simulink model "three_phase_dab"  (R2025a)
settings: Solver=ode1be  StartTime=0.0  StopTime=simlength  FixedStep=ts_sim  MaxStep=ts_sim
undefined symbols (not defined in the file or in its folder): Adrso, Aresd, Bresd, Cresd, Crso, dead_time, DThs_init, fPWM_INV, fPWM_ZVS, freq, frequency_grid, I_FS, Iout_dc_nom, ki_i_inv, ki_i_zvs, ki_pll, ki_v_inv, ki_v_zvs, kp_i_inv, kp_i_zvs, kp_pll, kp_v_inv, kp_v_zvs, Ldrso, magnitude, number_of_cells, Q, q1Kalman, q1kalman, q2Kalman, q2kalman, q3Kalman, rKalman, Rkalman, Tambient, tc, ts_dab, ts_inv, ts_zvs, tsample, V_FS, Vout_dc_nom, w, weigth
libraries: fl_lib x136, nesl_utility x98, ee_lib x21, cstblocks x7, lithium_ion_cell_lib x1, simulink x1, single_phase_transformer_lib x1
(part 2 of 7)

== system three_phase_dab/dab_modA/dab_ctrl/vi ctrl ==
  iout : Inport
  vout : Inport  Port=2
  vout_ref : Inport  Port=3
  Constant : Constant  Value=Iout_dc_nom
  Iout Ctrl : Subsystem
  Min : MinMax  Inputs=2
  To Workspace1 : ToWorkspace  VariableName=phase_ctrl_out_modA_sim  SampleTime=ts_zvs
      settings: MaxDataPoints=Ns_zvs
  To Workspace2 : ToWorkspace  VariableName=pid_ctrlv_out_modA_sim  SampleTime=ts_zvs
      settings: MaxDataPoints=Ns_zvs
  To Workspace3 : ToWorkspace  VariableName=pid_ctrli_out_modA_sim  SampleTime=ts_zvs
      settings: MaxDataPoints=Ns_zvs
  Unit Delay2 : UnitDelay  SampleTime=ts_zvs  HasFrameUpgradeWarning=on
  Vout Ctrl : Subsystem
  zvs_ctrl : Scope  NumInputPorts=2
      settings: SampleTime=tc  ActiveDisplayYMinimum=-1.16562  ActiveDisplayYMaximum=0.4906
  phase_displacement : Outport
  wires:
  Unit Delay2/1 -> phase_displacement/1, To Workspace1/1
  iout/1 -> Iout Ctrl/2(iout)
  vout_ref/1 -> Vout Ctrl/1(vout_ref)
  vout/1 -> Vout Ctrl/2(vout)
  Vout Ctrl/1(ctrlv_out) -> zvs_ctrl/1, Unit Delay2/1, To Workspace2/1  "u_ctrl_out"
  Constant/1 -> Iout Ctrl/1(iout_ref)
  Iout Ctrl/1(ctrli_out) -> zvs_ctrl/2, To Workspace3/1, Min/2  "i_ctrl_out"

== system three_phase_dab/dab_modA/dc//dc with galvanic isolation/stage-1 ==
  gate_commands : Inport
  Current Sensor : fl_lib/Electrical/Electrical Sensors/Current Sensor
  PS-Simulink Converter1 : nesl_utility/PS-Simulink Converter  PhysicalDomain=network_engine_domain  SubClassName=ps_output  LeftPortType=input  RightPortType=output  PseudoPeriodic=off  Frequencies=[]  VectorFormat=1-D array  Unit=A  AffineConversion=on
  h-bridge_thermal : Subsystem  Commented=on
  h-ideal : Subsystem  Commented=on
  h-mosfet : Subsystem
  uac_1(+) : PMIOPort  Side=Left
  uac_1(-) : PMIOPort  Port=2  Side=Left
  Udc(+) : PMIOPort  Port=3  Side=Right
  Udc(-) : PMIOPort  Port=4  Side=Right
  tag scope: dc_bus_terminal_current_inverter=global
  wires:
  gate_commands/1 -> h-mosfet/1(gate_commands)
  PS-Simulink Converter1/1 -> [dc_bus_terminal_current_inverter]  "idc"
  connections:
  h-mosfet/LConn1 -- uac_1(+)/RConn1
  h-mosfet/LConn2 -- uac_1(-)/RConn1
  h-mosfet/RConn2 -- Udc(-)/RConn1
  Current Sensor/LConn1 -- Udc(+)/RConn1
  h-mosfet/RConn1 -- Current Sensor/RConn2
  PS-Simulink Converter1/LConn1 -- Current Sensor/RConn1

== system three_phase_dab/dab_modA/dc//dc with galvanic isolation/stage-2 ==
  Current Sensor1 : fl_lib/Electrical/Electrical Sensors/Current Sensor
  PS-Simulink Converter2 : nesl_utility/PS-Simulink Converter  PhysicalDomain=network_engine_domain  SubClassName=ps_output  LeftPortType=input  RightPortType=output  PseudoPeriodic=off  Frequencies=[]  VectorFormat=1-D array  Unit=A  AffineConversion=on
  hf_trafo_center_tap_ss : Subsystem
  uac_1(+) : PMIOPort  Side=Left
  uac_2(+) : PMIOPort  Port=2  Side=Right
  uac_1(-) : PMIOPort  Port=3  Side=Left
  uac_2(-) : PMIOPort  Port=4  Side=Right
  connections:
  Current Sensor1/RConn2 -- uac_2(+)/RConn1
  PS-Simulink Converter2/LConn1 -- Current Sensor1/RConn1
  hf_trafo_center_tap_ss/LConn1 -- uac_1(+)/RConn1
  hf_trafo_center_tap_ss/RConn1 -- Current Sensor1/LConn1
  hf_trafo_center_tap_ss/LConn2 -- uac_1(-)/RConn1
  hf_trafo_center_tap_ss/RConn2 -- uac_2(-)/RConn1

== system three_phase_dab/dab_modA/dc//dc with galvanic isolation/stage-3 ==
  gate_commands : Inport
  CFu_dc : fl_lib/Electrical/Electrical Elements/Capacitor  c=CFu_dc F  r=RCFu_dc_internal Ohm  g=0 1/Ohm  i_specify=off  i_priority=None  i=0 A  i_nominal_specify=off  i_nominal_value=1  i_nominal_unit=A  v_specify=off  v_priority=None  v=0 V  v_nominal_specify=off  v_nominal_value=1  v_nominal_unit=V  vc_specify=off  vc_priority=High  vc=0 V  vc_nominal_specify=off  vc_nominal_value=1  vc_nominal_unit=V
  Current Sensor : fl_lib/Electrical/Electrical Sensors/Current Sensor
  Current Sensor2 : fl_lib/Electrical/Electrical Sensors/Current Sensor
  PS-Simulink Converter1 : nesl_utility/PS-Simulink Converter  PhysicalDomain=network_engine_domain  SubClassName=ps_output  LeftPortType=input  RightPortType=output  PseudoPeriodic=off  Frequencies=[]  VectorFormat=1-D array  Unit=A  AffineConversion=on
  PS-Simulink Converter6 : nesl_utility/PS-Simulink Converter  PhysicalDomain=network_engine_domain  SubClassName=ps_output  LeftPortType=input  RightPortType=output  PseudoPeriodic=off  Frequencies=[]  VectorFormat=1-D array  Unit=A  AffineConversion=on
  PS-Simulink Converter8 : nesl_utility/PS-Simulink Converter  PhysicalDomain=network_engine_domain  SubClassName=ps_output  LeftPortType=input  RightPortType=output  PseudoPeriodic=off  Frequencies=[]  VectorFormat=1-D array  Unit=V  AffineConversion=on
  Voltage Sensor4 : fl_lib/Electrical/Electrical Sensors/Voltage Sensor
  h-mosfet : Subsystem
  uac_1(+) : PMIOPort  Side=Left
  uac_1(-) : PMIOPort  Port=2  Side=Left
  udc(+) : PMIOPort  Port=3  Side=Right
  udc(-) : PMIOPort  Port=4  Side=Right
  tag scope: CFu_dc_current=global, CFu_dc_voltage=global
  wires:
  gate_commands/1 -> h-mosfet/1(gate_commands)
  PS-Simulink Converter6/1 -> [CFu_dc_current]  "i_Ls"
  PS-Simulink Converter8/1 -> [CFu_dc_voltage]  "CFu_dc_voltage"
  connections:
  h-mosfet/RConn1 -- Current Sensor/LConn1 -- CFu_dc/LConn1
  Voltage Sensor4/LConn1 -- udc(+)/RConn1 -- Current Sensor/RConn2
  h-mosfet/RConn2 -- Current Sensor2/RConn2 -- udc(-)/RConn1 -- Voltage Sensor4/RConn2
  h-mosfet/LConn2 -- uac_1(-)/RConn1
  h-mosfet/LConn1 -- uac_1(+)/RConn1
  Voltage Sensor4/RConn1 -- PS-Simulink Converter8/LConn1
  PS-Simulink Converter6/LConn1 -- Current Sensor2/RConn1
  CFu_dc/RConn1 -- Current Sensor2/LConn1
  Current Sensor/RConn1 -- PS-Simulink Converter1/LConn1

== system three_phase_dab/inverter_modA/single phase inverter/HBridgeIdeal ==
  gate_commands : Inport
  Bus Selector : BusSelector  OutputSignals=gate_cmd_Q1,gate_cmd_Q2,gate_cmd_Q3,gate_cmd_Q4
  Simulink-PS Converter{,1..3} (4 alike) : nesl_utility/Simulink-PS Converter  PhysicalDomain=network_engine_domain  SubClassName=ps_input  LeftPortType=input  RightPortType=output  PseudoPeriodic=off  Frequencies=[]  NoiseDistribution=none  NoiseParameters=[]  Unit=1  AffineConversion=on  FilteringAndDerivatives=provide  SimscapeFilterOrder=1  InputFilterTimeConstant=0.001  UdotUserProvided=0
  switch_1 : Subsystem
      settings: PortSchema="{\"entries\":[{\"content\":{\"sides\":[{\"content\":{\"connectorIds\":[\"LConn1\"]},\"type\":\"ConnectorPlacement.EquallySpacedRectSide\",\"uuid\":\"9277da8d-d460-43e6-8478-dd662f15d226\"},{\"content\":{\"connectorIds\":[],\"side\":\"RIGHT\"},\"type\":\"ConnectorPlacement.EquallySpacedRectSide\",\"uuid\":\"a7ece396-f1d9-4f4f-a05b-db1fc65d6e1d\"},{\"content\":{\"connectorIds\":[\"LConn2\"],\"side\":\"TOP\"},\"type\":\"ConnectorPlacement.EquallySpacedRectSide\",\"uuid\":\"fdd70777-e9cf-4317-afb6-cae87f75d5b0\"},{\"content\":{\"connectorIds\":[\"RConn1\"],\"side\":\"BOTTOM\"},\"type\":\"ConnectorPlacement.EquallySpacedRectSide\",\"uuid\":\"2353ed68-b1a1-4775-9ca9-31e268d5443b\"}]},\"type\":\"ConnectorPlacement.EquallySpacedConnector\",\"uuid\":\"d5479f4c-4e65-4791-adcb-73df11f88590\"}],\"packageUris\":[\"http://schema.mathworks.com/mf0/Connector/R2020b\"],\"version\":\"1.0\"}"
  switch_2 : Subsystem
      settings: PortSchema="{\"entries\":[{\"content\":{\"sides\":[{\"content\":{\"connectorIds\":[\"LConn1\"]},\"type\":\"ConnectorPlacement.EquallySpacedRectSide\",\"uuid\":\"9277da8d-d460-43e6-8478-dd662f15d226\"},{\"content\":{\"connectorIds\":[],\"side\":\"RIGHT\"},\"type\":\"ConnectorPlacement.EquallySpacedRectSide\",\"uuid\":\"a7ece396-f1d9-4f4f-a05b-db1fc65d6e1d\"},{\"content\":{\"connectorIds\":[\"LConn2\"],\"side\":\"TOP\"},\"type\":\"ConnectorPlacement.EquallySpacedRectSide\",\"uuid\":\"fdd70777-e9cf-4317-afb6-cae87f75d5b0\"},{\"content\":{\"connectorIds\":[\"RConn1\"],\"side\":\"BOTTOM\"},\"type\":\"ConnectorPlacement.EquallySpacedRectSide\",\"uuid\":\"2353ed68-b1a1-4775-9ca9-31e268d5443b\"}]},\"type\":\"ConnectorPlacement.EquallySpacedConnector\",\"uuid\":\"d5479f4c-4e65-4791-adcb-73df11f88590\"}],\"packageUris\":[\"http://schema.mathworks.com/mf0/Connector/R2020b\"],\"version\":\"1.0\"}"
  switch_3 : Subsystem
      settings: PortSchema="{\"entries\":[{\"content\":{\"sides\":[{\"content\":{\"connectorIds\":[\"LConn1\"]},\"type\":\"ConnectorPlacement.EquallySpacedRectSide\",\"uuid\":\"9277da8d-d460-43e6-8478-dd662f15d226\"},{\"content\":{\"connectorIds\":[],\"side\":\"RIGHT\"},\"type\":\"ConnectorPlacement.EquallySpacedRectSide\",\"uuid\":\"a7ece396-f1d9-4f4f-a05b-db1fc65d6e1d\"},{\"content\":{\"connectorIds\":[\"LConn2\"],\"side\":\"TOP\"},\"type\":\"ConnectorPlacement.EquallySpacedRectSide\",\"uuid\":\"fdd70777-e9cf-4317-afb6-cae87f75d5b0\"},{\"content\":{\"connectorIds\":[\"RConn1\"],\"side\":\"BOTTOM\"},\"type\":\"ConnectorPlacement.EquallySpacedRectSide\",\"uuid\":\"2353ed68-b1a1-4775-9ca9-31e268d5443b\"}]},\"type\":\"ConnectorPlacement.EquallySpacedConnector\",\"uuid\":\"d5479f4c-4e65-4791-adcb-73df11f88590\"}],\"packageUris\":[\"http://schema.mathworks.com/mf0/Connector/R2020b\"],\"version\":\"1.0\"}"
  switch_4 : Subsystem
      settings: PortSchema="{\"entries\":[{\"content\":{\"sides\":[{\"content\":{\"connectorIds\":[\"LConn1\"]},\"type\":\"ConnectorPlacement.EquallySpacedRectSide\",\"uuid\":\"9277da8d-d460-43e6-8478-dd662f15d226\"},{\"content\":{\"connectorIds\":[],\"side\":\"RIGHT\"},\"type\":\"ConnectorPlacement.EquallySpacedRectSide\",\"uuid\":\"a7ece396-f1d9-4f4f-a05b-db1fc65d6e1d\"},{\"content\":{\"connectorIds\":[\"LConn2\"],\"side\":\"TOP\"},\"type\":\"ConnectorPlacement.EquallySpacedRectSide\",\"uuid\":\"fdd70777-e9cf-4317-afb6-cae87f75d5b0\"},{\"content\":{\"connectorIds\":[\"RConn1\"],\"side\":\"BOTTOM\"},\"type\":\"ConnectorPlacement.EquallySpacedRectSide\",\"uuid\":\"2353ed68-b1a1-4775-9ca9-31e268d5443b\"}]},\"type\":\"ConnectorPlacement.EquallySpacedConnector\",\"uuid\":\"d5479f4c-4e65-4791-adcb-73df11f88590\"}],\"packageUris\":[\"http://schema.mathworks.com/mf0/Connector/R2020b\"],\"version\":\"1.0\"}"
  C : PMIOPort  Side=Left
  E : PMIOPort  Port=2  Side=Right
  C1 : PMIOPort  Port=3  Side=Right
  E1 : PMIOPort  Port=4  Side=Left
  wires:
  [gate_Q3] -> Simulink-PS Converter2/1
  Bus Selector/2 -> [gate_Q2]  "<gate_cmd_Q2>"
  Bus Selector/1 -> [gate_Q1]  "<gate_cmd_Q1>"
  Bus Selector/3 -> [gate_Q3]  "<gate_cmd_Q3>"
  [gate_Q4] -> Simulink-PS Converter3/1
  [gate_Q2] -> Simulink-PS Converter1/1
  [gate_Q1] -> Simulink-PS Converter/1
  Bus Selector/4 -> [gate_Q4]  "<gate_cmd_Q4>"
  gate_commands/1 -> Bus Selector/1
  connections:
  switch_1/LConn1 -- Simulink-PS Converter/RConn1
  switch_3/LConn2 -- C/RConn1 -- switch_1/LConn2
  switch_4/RConn1 -- E1/RConn1 -- switch_2/RConn1
  switch_2/LConn2 -- switch_1/RConn1 -- E/RConn1
  switch_3/LConn1 -- Simulink-PS Converter2/RConn1
  switch_3/RConn1 -- switch_4/LConn2 -- C1/RConn1
  switch_2/LConn1 -- Simulink-PS Converter1/RConn1
  switch_4/LConn1 -- Simulink-PS Converter3/RConn1

== system three_phase_dab/inverter_modA/single phase inverter/HBridgeMosfet ==
  gate_commands : Inport
  Bus Selector : BusSelector  OutputSignals=gate_cmd_Q1,gate_cmd_Q2,gate_cmd_Q3,gate_cmd_Q4
  Simulink-PS Converter{,1..3} (4 alike) : nesl_utility/Simulink-PS Converter  PhysicalDomain=network_engine_domain  SubClassName=ps_input  LeftPortType=input  RightPortType=output  PseudoPeriodic=off  Frequencies=[]  NoiseDistribution=none  NoiseParameters=[]  Unit=V  AffineConversion=off  FilteringAndDerivatives=provide  SimscapeFilterOrder=1  InputFilterTimeConstant=0.001  UdotUserProvided=0
  mosfet_1 : Subsystem
      settings: PortSchema="{\"entries\":[{\"content\":{\"sides\":[{\"content\":{\"connectorIds\":[\"LConn1\"]},\"type\":\"ConnectorPlacement.EquallySpacedRectSide\",\"uuid\":\"9277da8d-d460-43e6-8478-dd662f15d226\"},{\"content\":{\"connectorIds\":[],\"side\":\"RIGHT\"},\"type\":\"ConnectorPlacement.EquallySpacedRectSide\",\"uuid\":\"a7ece396-f1d9-4f4f-a05b-db1fc65d6e1d\"},{\"content\":{\"connectorIds\":[\"LConn2\"],\"side\":\"TOP\"},\"type\":\"ConnectorPlacement.EquallySpacedRectSide\",\"uuid\":\"fdd70777-e9cf-4317-afb6-cae87f75d5b0\"},{\"content\":{\"connectorIds\":[\"RConn1\"],\"side\":\"BOTTOM\"},\"type\":\"ConnectorPlacement.EquallySpacedRectSide\",\"uuid\":\"2353ed68-b1a1-4775-9ca9-31e268d5443b\"}]},\"type\":\"ConnectorPlacement.EquallySpacedConnector\",\"uuid\":\"d5479f4c-4e65-4791-adcb-73df11f88590\"}],\"packageUris\":[\"http://schema.mathworks.com/mf0/Connector/R2020b\"],\"version\":\"1.0\"}"
  mosfet_2 : Subsystem
      settings: PortSchema="{\"entries\":[{\"content\":{\"sides\":[{\"content\":{\"connectorIds\":[\"LConn1\"]},\"type\":\"ConnectorPlacement.EquallySpacedRectSide\",\"uuid\":\"9277da8d-d460-43e6-8478-dd662f15d226\"},{\"content\":{\"connectorIds\":[],\"side\":\"RIGHT\"},\"type\":\"ConnectorPlacement.EquallySpacedRectSide\",\"uuid\":\"a7ece396-f1d9-4f4f-a05b-db1fc65d6e1d\"},{\"content\":{\"connectorIds\":[\"LConn2\"],\"side\":\"TOP\"},\"type\":\"ConnectorPlacement.EquallySpacedRectSide\",\"uuid\":\"fdd70777-e9cf-4317-afb6-cae87f75d5b0\"},{\"content\":{\"connectorIds\":[\"RConn1\"],\"side\":\"BOTTOM\"},\"type\":\"ConnectorPlacement.EquallySpacedRectSide\",\"uuid\":\"2353ed68-b1a1-4775-9ca9-31e268d5443b\"}]},\"type\":\"ConnectorPlacement.EquallySpacedConnector\",\"uuid\":\"d5479f4c-4e65-4791-adcb-73df11f88590\"}],\"packageUris\":[\"http://schema.mathworks.com/mf0/Connector/R2020b\"],\"version\":\"1.0\"}"
  mosfet_3 : Subsystem
      settings: PortSchema="{\"entries\":[{\"content\":{\"sides\":[{\"content\":{\"connectorIds\":[\"LConn1\"]},\"type\":\"ConnectorPlacement.EquallySpacedRectSide\",\"uuid\":\"9277da8d-d460-43e6-8478-dd662f15d226\"},{\"content\":{\"connectorIds\":[],\"side\":\"RIGHT\"},\"type\":\"ConnectorPlacement.EquallySpacedRectSide\",\"uuid\":\"a7ece396-f1d9-4f4f-a05b-db1fc65d6e1d\"},{\"content\":{\"connectorIds\":[\"LConn2\"],\"side\":\"TOP\"},\"type\":\"ConnectorPlacement.EquallySpacedRectSide\",\"uuid\":\"fdd70777-e9cf-4317-afb6-cae87f75d5b0\"},{\"content\":{\"connectorIds\":[\"RConn1\"],\"side\":\"BOTTOM\"},\"type\":\"ConnectorPlacement.EquallySpacedRectSide\",\"uuid\":\"2353ed68-b1a1-4775-9ca9-31e268d5443b\"}]},\"type\":\"ConnectorPlacement.EquallySpacedConnector\",\"uuid\":\"d5479f4c-4e65-4791-adcb-73df11f88590\"}],\"packageUris\":[\"http://schema.mathworks.com/mf0/Connector/R2020b\"],\"version\":\"1.0\"}"
  mosfet_4 : Subsystem
      settings: PortSchema="{\"entries\":[{\"content\":{\"sides\":[{\"content\":{\"connectorIds\":[\"LConn1\"]},\"type\":\"ConnectorPlacement.EquallySpacedRectSide\",\"uuid\":\"9277da8d-d460-43e6-8478-dd662f15d226\"},{\"content\":{\"connectorIds\":[],\"side\":\"RIGHT\"},\"type\":\"ConnectorPlacement.EquallySpacedRectSide\",\"uuid\":\"a7ece396-f1d9-4f4f-a05b-db1fc65d6e1d\"},{\"content\":{\"connectorIds\":[\"LConn2\"],\"side\":\"TOP\"},\"type\":\"ConnectorPlacement.EquallySpacedRectSide\",\"uuid\":\"fdd70777-e9cf-4317-afb6-cae87f75d5b0\"},{\"content\":{\"connectorIds\":[\"RConn1\"],\"side\":\"BOTTOM\"},\"type\":\"ConnectorPlacement.EquallySpacedRectSide\",\"uuid\":\"2353ed68-b1a1-4775-9ca9-31e268d5443b\"}]},\"type\":\"ConnectorPlacement.EquallySpacedConnector\",\"uuid\":\"d5479f4c-4e65-4791-adcb-73df11f88590\"}],\"packageUris\":[\"http://schema.mathworks.com/mf0/Connector/R2020b\"],\"version\":\"1.0\"}"
  C : PMIOPort  Side=Left
  E : PMIOPort  Port=2  Side=Right
  C1 : PMIOPort  Port=3  Side=Right
  E1 : PMIOPort  Port=4  Side=Left
  wires:
  [gate_Q3] -> Simulink-PS Converter2/1
  Bus Selector/2 -> [gate_Q2]  "<gate_cmd_Q2>"
  Bus Selector/1 -> [gate_Q1]  "<gate_cmd_Q1>"
  Bus Selector/3 -> [gate_Q3]  "<gate_cmd_Q3>"
  [gate_Q4] -> Simulink-PS Converter3/1
  [gate_Q2] -> Simulink-PS Converter1/1
  [gate_Q1] -> Simulink-PS Converter/1
  Bus Selector/4 -> [gate_Q4]  "<gate_cmd_Q4>"
  gate_commands/1 -> Bus Selector/1
  connections:
  mosfet_1/LConn1 -- Simulink-PS Converter/RConn1
  C/RConn1 -- mosfet_3/LConn2 -- mosfet_1/LConn2
  E1/RConn1 -- mosfet_4/RConn1 -- mosfet_2/RConn1
  E/RConn1 -- mosfet_2/LConn2 -- mosfet_1/RConn1
  mosfet_3/LConn1 -- Simulink-PS Converter2/RConn1
  C1/RConn1 -- mosfet_4/LConn2 -- mosfet_3/RConn1
  mosfet_2/LConn1 -- Simulink-PS Converter1/RConn1
  mosfet_4/LConn1 -- Simulink-PS Converter3/RConn1

== system three_phase_dab/inverter_modA/single phase inverter/HBridgeThermal ==
  gate_commands : Inport
  Bus Selector : BusSelector  OutputSignals=gate_cmd_Q1,gate_cmd_Q2,gate_cmd_Q3,gate_cmd_Q4
  Simulink-PS Converter{,1..3} (4 alike) : nesl_utility/Simulink-PS Converter  PhysicalDomain=network_engine_domain  SubClassName=ps_input  LeftPortType=input  RightPortType=output  PseudoPeriodic=off  Frequencies=[]  NoiseDistribution=none  NoiseParameters=[]  Unit=V  AffineConversion=off  FilteringAndDerivatives=provide  SimscapeFilterOrder=1  InputFilterTimeConstant=0.001  UdotUserProvided=0
  mosfet_thermal_1 : Subsystem
      settings: PortSchema="{\"entries\":[{\"content\":{\"sides\":[{\"content\":{\"connectorIds\":[\"LConn1\"]},\"type\":\"ConnectorPlacement.EquallySpacedRectSide\",\"uuid\":\"9277da8d-d460-43e6-8478-dd662f15d226\"},{\"content\":{\"connectorIds\":[],\"side\":\"RIGHT\"},\"type\":\"ConnectorPlacement.EquallySpacedRectSide\",\"uuid\":\"a7ece396-f1d9-4f4f-a05b-db1fc65d6e1d\"},{\"content\":{\"connectorIds\":[\"LConn2\"],\"side\":\"TOP\"},\"type\":\"ConnectorPlacement.EquallySpacedRectSide\",\"uuid\":\"fdd70777-e9cf-4317-afb6-cae87f75d5b0\"},{\"content\":{\"connectorIds\":[\"RConn1\"],\"side\":\"BOTTOM\"},\"type\":\"ConnectorPlacement.EquallySpacedRectSide\",\"uuid\":\"2353ed68-b1a1-4775-9ca9-31e268d5443b\"}]},\"type\":\"ConnectorPlacement.EquallySpacedConnector\",\"uuid\":\"d5479f4c-4e65-4791-adcb-73df11f88590\"}],\"packageUris\":[\"http://schema.mathworks.com/mf0/Connector/R2020b\"],\"version\":\"1.0\"}"
  mosfet_thermal_2 : Subsystem
      settings: PortSchema="{\"entries\":[{\"content\":{\"sides\":[{\"content\":{\"connectorIds\":[\"LConn1\"]},\"type\":\"ConnectorPlacement.EquallySpacedRectSide\",\"uuid\":\"9277da8d-d460-43e6-8478-dd662f15d226\"},{\"content\":{\"connectorIds\":[],\"side\":\"RIGHT\"},\"type\":\"ConnectorPlacement.EquallySpacedRectSide\",\"uuid\":\"a7ece396-f1d9-4f4f-a05b-db1fc65d6e1d\"},{\"content\":{\"connectorIds\":[\"LConn2\"],\"side\":\"TOP\"},\"type\":\"ConnectorPlacement.EquallySpacedRectSide\",\"uuid\":\"fdd70777-e9cf-4317-afb6-cae87f75d5b0\"},{\"content\":{\"connectorIds\":[\"RConn1\"],\"side\":\"BOTTOM\"},\"type\":\"ConnectorPlacement.EquallySpacedRectSide\",\"uuid\":\"2353ed68-b1a1-4775-9ca9-31e268d5443b\"}]},\"type\":\"ConnectorPlacement.EquallySpacedConnector\",\"uuid\":\"d5479f4c-4e65-4791-adcb-73df11f88590\"}],\"packageUris\":[\"http://schema.mathworks.com/mf0/Connector/R2020b\"],\"version\":\"1.0\"}"
  mosfet_thermal_3 : Subsystem
      settings: PortSchema="{\"entries\":[{\"content\":{\"sides\":[{\"content\":{\"connectorIds\":[\"LConn1\"]},\"type\":\"ConnectorPlacement.EquallySpacedRectSide\",\"uuid\":\"9277da8d-d460-43e6-8478-dd662f15d226\"},{\"content\":{\"connectorIds\":[],\"side\":\"RIGHT\"},\"type\":\"ConnectorPlacement.EquallySpacedRectSide\",\"uuid\":\"a7ece396-f1d9-4f4f-a05b-db1fc65d6e1d\"},{\"content\":{\"connectorIds\":[\"LConn2\"],\"side\":\"TOP\"},\"type\":\"ConnectorPlacement.EquallySpacedRectSide\",\"uuid\":\"fdd70777-e9cf-4317-afb6-cae87f75d5b0\"},{\"content\":{\"connectorIds\":[\"RConn1\"],\"side\":\"BOTTOM\"},\"type\":\"ConnectorPlacement.EquallySpacedRectSide\",\"uuid\":\"2353ed68-b1a1-4775-9ca9-31e268d5443b\"}]},\"type\":\"ConnectorPlacement.EquallySpacedConnector\",\"uuid\":\"d5479f4c-4e65-4791-adcb-73df11f88590\"}],\"packageUris\":[\"http://schema.mathworks.com/mf0/Connector/R2020b\"],\"version\":\"1.0\"}"
  mosfet_thermal_4 : Subsystem
      settings: PortSchema="{\"entries\":[{\"content\":{\"sides\":[{\"content\":{\"connectorIds\":[\"LConn1\"]},\"type\":\"ConnectorPlacement.EquallySpacedRectSide\",\"uuid\":\"9277da8d-d460-43e6-8478-dd662f15d226\"},{\"content\":{\"connectorIds\":[],\"side\":\"RIGHT\"},\"type\":\"ConnectorPlacement.EquallySpacedRectSide\",\"uuid\":\"a7ece396-f1d9-4f4f-a05b-db1fc65d6e1d\"},{\"content\":{\"connectorIds\":[\"LConn2\"],\"side\":\"TOP\"},\"type\":\"ConnectorPlacement.EquallySpacedRectSide\",\"uuid\":\"fdd70777-e9cf-4317-afb6-cae87f75d5b0\"},{\"content\":{\"connectorIds\":[\"RConn1\"],\"side\":\"BOTTOM\"},\"type\":\"ConnectorPlacement.EquallySpacedRectSide\",\"uuid\":\"2353ed68-b1a1-4775-9ca9-31e268d5443b\"}]},\"type\":\"ConnectorPlacement.EquallySpacedConnector\",\"uuid\":\"d5479f4c-4e65-4791-adcb-73df11f88590\"}],\"packageUris\":[\"http://schema.mathworks.com/mf0/Connector/R2020b\"],\"version\":\"1.0\"}"
  C : PMIOPort  Side=Left
  E : PMIOPort  Port=2  Side=Right
  C1 : PMIOPort  Port=3  Side=Right
  E1 : PMIOPort  Port=4  Side=Left
  wires:
  gate_commands/1 -> Bus Selector/1
  Bus Selector/4 -> [gate_Q4]  "<gate_cmd_Q4>"
  [gate_Q1] -> Simulink-PS Converter/1
  [gate_Q2] -> Simulink-PS Converter1/1
  [gate_Q4] -> Simulink-PS Converter3/1
  Bus Selector/3 -> [gate_Q3]  "<gate_cmd_Q3>"
  Bus Selector/1 -> [gate_Q1]  "<gate_cmd_Q1>"
  Bus Selector/2 -> [gate_Q2]  "<gate_cmd_Q2>"
  [gate_Q3] -> Simulink-PS Converter2/1
  connections:
  mosfet_thermal_4/LConn1 -- Simulink-PS Converter3/RConn1
  mosfet_thermal_2/LConn1 -- Simulink-PS Converter1/RConn1
  C1/RConn1 -- mosfet_thermal_4/LConn2 -- mosfet_thermal_3/RConn1
  mosfet_thermal_3/LConn1 -- Simulink-PS Converter2/RConn1
  E/RConn1 -- mosfet_thermal_1/RConn1 -- mosfet_thermal_2/LConn2
  E1/RConn1 -- mosfet_thermal_4/RConn1 -- mosfet_thermal_2/RConn1
  mosfet_thermal_1/LConn2 -- mosfet_thermal_3/LConn2 -- C/RConn1
  mosfet_thermal_1/LConn1 -- Simulink-PS Converter/RConn1

== system three_phase_dab/inverter_modA/single phase inverter control/acquisition_and_scaling_current ==
  in : Inport
  1/Ti5 : Gain  Gain=1/I_FS  SaturateOnIntegerOverflow=on  OutDataTypeStr=Inherit: Same as input  ParamDataTypeStr=Inherit: Same as input
  Unit Delay4 : UnitDelay  SampleTime=ts_inv  HasFrameUpgradeWarning=on
  Zero-Order Hold1 : ZeroOrderHold  SampleTime=ts_inv
  out : Outport
  wires:
  in/1 -> Zero-Order Hold1/1
  1/Ti5/1 -> Unit Delay4/1
  Zero-Order Hold1/1 -> 1/Ti5/1
  Unit Delay4/1 -> out/1

== system three_phase_dab/inverter_modA/single phase inverter control/acquisition_and_scaling_voltage ==
  in : Inport
  1/Ti1 : Gain  Gain=1/V_FS  SaturateOnIntegerOverflow=on  OutDataTypeStr=Inherit: Same as input  ParamDataTypeStr=Inherit: Same as input
  Unit Delay4 : UnitDelay  SampleTime=ts_inv  HasFrameUpgradeWarning=on
  Zero-Order Hold2 : ZeroOrderHold  SampleTime=ts_inv
  out : Outport
  wires:
  1/Ti1/1 -> Unit Delay4/1
  Zero-Order Hold2/1 -> 1/Ti1/1
  Unit Delay4/1 -> out/1
  in/1 -> Zero-Order Hold2/1

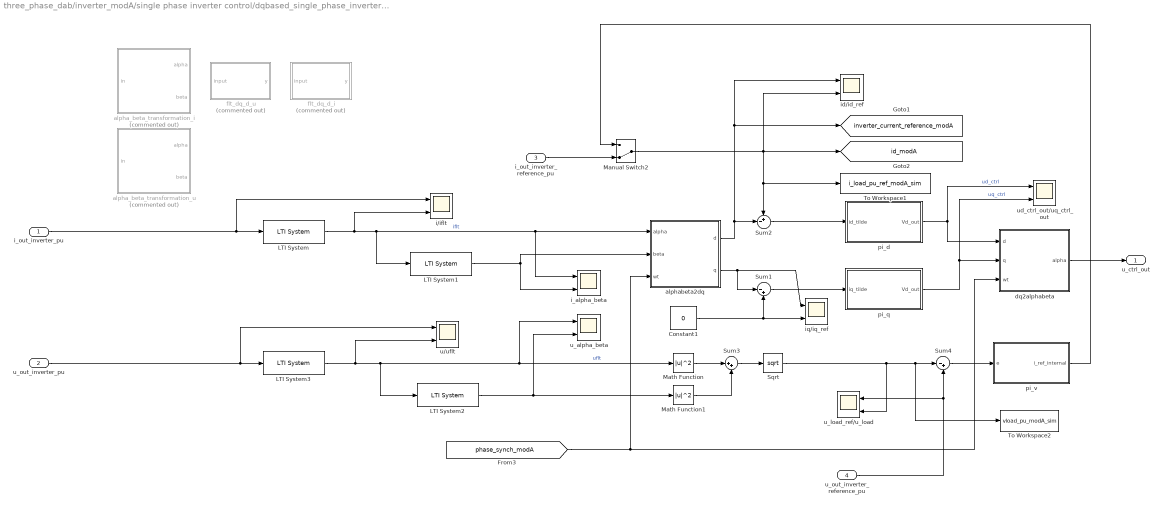
== system three_phase_dab/inverter_modA/single phase inverter control/dqbased_single_phase_inverter_ctrl ==
  i_out_inverter_pu : Inport
  u_out_inverter_pu : Inport  Port=2
  i_out_inverter_reference_pu : Inport  Port=3
  u_out_inverter_reference_pu : Inport  Port=4
  Constant1 : Constant  Value=0
  LTI System : cstblocks/LTI System  sys=resd_tf  IC=[]  PadeOrder=0
  LTI System1 : cstblocks/LTI System  sys=flt_dq_d  IC=[]  PadeOrder=0
  LTI System2 : cstblocks/LTI System  sys=flt_dq_d  IC=[]  PadeOrder=0
  LTI System3 : cstblocks/LTI System  sys=resd_tf  IC=[]  PadeOrder=0
  Manual Switch2 : ManualSwitch  CurrentSetting=0
  Math Function : Math  Operator=magnitude^2
  Math Function1 : Math  Operator=magnitude^2
  Sqrt : Sqrt
  Sum1 : Sum  Inputs=|-+
  Sum2 : Sum  Inputs=+-|
  Sum3 : Sum  Inputs=|++
  Sum4 : Sum  Inputs=|-+
  To Workspace1 : ToWorkspace  VariableName=i_load_pu_ref_modA_sim  SampleTime=ts_inv
      settings: MaxDataPoints=Ns_inv
  To Workspace2 : ToWorkspace  VariableName=vload_pu_modA_sim  SampleTime=ts_inv
      settings: MaxDataPoints=Ns_inv
  alpha_beta_transformation_i : Subsystem  Commented=on
  alpha_beta_transformation_u : Subsystem  Commented=on
  alphabeta2dq : Subsystem
  dq2alphabeta : Subsystem
  flt_dq_d_i : MATLAB Function  Commented=on  TreatAsAtomicUnit=on  SystemSampleTime=ts_inv
  flt_dq_d_u : MATLAB Function  Commented=on  TreatAsAtomicUnit=on  SystemSampleTime=ts_inv
  i/iflt : Scope  NumInputPorts=2
      settings: ActiveDisplayYMinimum=-56.02129  ActiveDisplayYMaximum=332.90712  DataLoggingVariableName=ScopeData3
  i_alpha_beta : Scope  NumInputPorts=2
      settings: ActiveDisplayYMinimum=-0.58436  ActiveDisplayYMaximum=0.5476  DataLoggingVariableName=ScopeData2
  id/id_ref : Scope  NumInputPorts=2
      settings: SampleTime=tc  ActiveDisplayYMinimum=-166.58726  ActiveDisplayYMaximum=107.66374  DataLoggingVariableName=ScopeData2
  iq/iq_ref : Scope  NumInputPorts=2
      settings: SampleTime=tc  ActiveDisplayYMinimum=-455.06009  ActiveDisplayYMaximum=206.06184  DataLoggingVariableName=ScopeData3
  pi_d : Subsystem
  pi_q : Subsystem
  pi_v : Subsystem
  u/uflt : Scope  NumInputPorts=2
      settings: ActiveDisplayYMinimum=-0.91252  ActiveDisplayYMaximum=0.91352  DataLoggingVariableName=ScopeData4
  u_alpha_beta : Scope  NumInputPorts=2
      settings: ActiveDisplayYMinimum=-0.39479  ActiveDisplayYMaximum=0.39668
  u_load_ref/u_load : Scope  NumInputPorts=2
      settings: ActiveDisplayYMinimum=-4.64085  ActiveDisplayYMaximum=41.76761
  ud_ctrl_out/uq_ctrl_out : Scope  NumInputPorts=2
      settings: ActiveDisplayYMinimum=-1.25  ActiveDisplayYMaximum=1.25  DataLoggingVariableName=ScopeData2
  u_ctrl_out : Outport
  tag scope: id_modA=global, inverter_current_reference_modA=global
  wires:
  alphabeta2dq/1("d ") -> Sum2/2, id/id_ref/1, [inverter_current_reference_modA]
  Sqrt/1 -> u_load_ref/u_load/2, To Workspace2/1, Sum4/1
  i_out_inverter_pu/1 -> LTI System/1, i/iflt/1
  Math Function/1 -> Sum3/1
  LTI System1/1 -> alphabeta2dq/2(beta), i_alpha_beta/2
  LTI System/1 -> i/iflt/2, LTI System1/1, alphabeta2dq/1(alpha), i_alpha_beta/1  "iflt"
  [phase_synch_modA] -> alphabeta2dq/3(wt), dq2alphabeta/3(wt)
  pi_q/1(Vd_out) -> dq2alphabeta/2(q), ud_ctrl_out/uq_ctrl_out/2  "uq_ctrl"
  alphabeta2dq/2("q ") -> Sum1/1, iq/iq_ref/1
  Sum4/1 -> pi_v/1(e)
  pi_d/1(Vd_out) -> ud_ctrl_out/uq_ctrl_out/1, dq2alphabeta/1(d)  "ud_ctrl"
  Manual Switch2/1 -> id/id_ref/2, [id_modA], Sum2/1, To Workspace1/1
  i_out_inverter_reference_pu/1 -> Manual Switch2/2
  LTI System3/1 -> Math Function/1, u_alpha_beta/1, LTI System2/1, u/uflt/2  "uflt"
  Sum1/1 -> pi_q/1(iq_tilde)
  Math Function1/1 -> Sum3/2
  Sum2/1 -> pi_d/1(id_tilde)
  LTI System2/1 -> u_alpha_beta/2, Math Function1/1
  Constant1/1 -> iq/iq_ref/2, Sum1/2
  u_out_inverter_pu/1 -> LTI System3/1, u/uflt/1
  pi_v/1(i_ref_internal) -> Manual Switch2/1
  dq2alphabeta/1(alpha) -> u_ctrl_out/1
  Sum3/1 -> Sqrt/1
  u_out_inverter_reference_pu/1 -> u_load_ref/u_load/1, Sum4/2

== system three_phase_dab/inverter_modA/single phase inverter control/pwm ==
  vout : Inport
  Constant : Constant  Value=0
  Constant{1..4} (4 alike) : Constant
  Gain1 : Gain  Gain=1/2
  Gain2 : Gain
  Gain3 : Gain  Gain=1/2
  Gain4 : Gain  Gain=-1
  PWM generator 1 : Subsystem  mask{f=fPWM_INV, m_up=0.98, m_low=0.02, dead_time=dead_time, pos_cmd_gate=15, neg_cmd_gate=-10, polarity=-1}
      mask prompts: f "Frequency (Hz)"; m_up "Max Input Modulation Value"; m_low "Min Input Modulation Value"; dead_time "Dead Time (s)"; pos_cmd_gate "Positive Gate Voltage (V)"; neg_cmd_gate "Negative Gate Voltage (V)"; polarity "Polarity (pu)"
  PWM generator 2 : Subsystem  mask{f=fPWM_INV, m_up=0.98, m_low=0.02, dead_time=dead_time, pos_cmd_gate=15, neg_cmd_gate=-10, polarity=-1}
      mask prompts: f "Frequency (Hz)"; m_up "Max Input Modulation Value"; m_low "Min Input Modulation Value"; dead_time "Dead Time (s)"; pos_cmd_gate "Positive Gate Voltage (V)"; neg_cmd_gate "Negative Gate Voltage (V)"; polarity "Polarity (pu)"
  Product{,1..3} (4 alike) : Product
  Sum : Sum  Inputs=|++
  Sum1 : Sum  Inputs=|++
  m1_top : Outport
  m1_bottom : Outport  Port=2
  m2_top : Outport  Port=3
  m2_bottom : Outport  Port=4
  wires:
  Constant/1 -> PWM generator 2/2(phase), PWM generator 1/2(phase)
  Constant1/1 -> PWM generator 2/3(polarity_input), PWM generator 1/3(polarity_input)
  Gain2/1 -> Sum/1
  Sum/1 -> Gain1/1
  Constant2/1 -> Sum/2
  Gain1/1 -> PWM generator 1/1(m_index)
  Constant3/1 -> Sum1/2
  Sum1/1 -> Gain3/1
  Gain4/1 -> Sum1/1
  Gain3/1 -> PWM generator 2/1(m_index)
  vout/1 -> Gain4/1, Gain2/1
  PWM generator 1/1(m1) -> Product/1  "gate_cmd_Q1"
  PWM generator 1/2(m2) -> Product1/1  "gate_cmd_Q2"
  PWM generator 2/1(m1) -> Product2/1  "gate_cmd_Q3"
  PWM generator 2/2(m2) -> Product3/1  "gate_cmd_Q4"
  Product/1 -> m1_top/1  "gate_cmd_Q1"
  Product1/1 -> m1_bottom/1  "gate_cmd_Q2"
  Product2/1 -> m2_top/1  "gate_cmd_Q3"
  Product3/1 -> m2_bottom/1  "gate_cmd_Q4"
  Constant4/1 -> Product3/2, Product2/2, Product1/2, Product/2

== system three_phase_dab/inverter_modA/single phase inverter control/references_generator ==
  1/Ti2 : Gain  Gain=1/V_FS  SaturateOnIntegerOverflow=on  OutDataTypeStr=Inherit: Same as input  ParamDataTypeStr=Inherit: Same as input
  1/Ti4 : Gain  Gain=1/I_FS  SaturateOnIntegerOverflow=on  OutDataTypeStr=Inherit: Same as input  ParamDataTypeStr=Inherit: Same as input
  Rate Limiter : RateLimiter  SampleTimeMode=inherited
  Rate Limiter1 : RateLimiter  SampleTimeMode=inherited
  Zero-Order Hold3 : ZeroOrderHold  SampleTime=ts_inv
  Zero-Order Hold4 : ZeroOrderHold  SampleTime=ts_inv
  i_out_inverter_reference : Step  Time=0.75  After=-I_FS  SampleTime=0
  u_out_inverter_reference : Step  Time=0.5  After=230*sqrt(2)  SampleTime=0
  i_out_inverter_reference_pu : Outport
  u_out_inverter_reference_pu : Outport  Port=2
  wires:
  Zero-Order Hold3/1 -> i_out_inverter_reference_pu/1
  1/Ti4/1 -> Rate Limiter1/1
  1/Ti2/1 -> Rate Limiter/1
  Rate Limiter/1 -> Zero-Order Hold4/1
  Zero-Order Hold4/1 -> u_out_inverter_reference_pu/1
  Rate Limiter1/1 -> Zero-Order Hold3/1
  i_out_inverter_reference/1 -> 1/Ti4/1
  u_out_inverter_reference/1 -> 1/Ti2/1

== system three_phase_dab/inverter_modA/single phase inverter control/rpi_based_single_phase_inverter_ctrl ==
  i_out_inverter_pu : Inport
  u_out_inverter_pu : Inport  Port=2
  i_out_inverter_reference_pu : Inport  Port=3
  u_out_inverter_reference_pu : Inport  Port=4
  Manual Switch2 : ManualSwitch
  current_reference_generation : Subsystem
  is/is_ref : Scope  NumInputPorts=2
      settings: SampleTime=tc  ActiveDisplayYMinimum=-1.00771  ActiveDisplayYMaximum=1.0071  DataLoggingVariableName=ScopeData2
  load_current_control : Subsystem
  load_voltage_control : Subsystem
  u_ctrl_out : Outport
  tag scope: i_out_inverter_pu=global, i_out_inverter_pu_ref=global, id_inv_pu_ref=global
  wires:
  i_out_inverter_pu/1 -> load_current_control/2(i_out_inverter_pu), [i_out_inverter_pu], is/is_ref/1  "i_out_inverter_pu"
  load_current_control/1(u_ctrl_out) -> u_ctrl_out/1  "u_ctrl_out"
  current_reference_generation/1(phase_ref) -> [i_out_inverter_pu_ref], is/is_ref/2, load_current_control/1(i_out_inverter_reference_pu)  "i_out_inverter_pu_ref"
  Manual Switch2/1 -> [id_inv_pu_ref], current_reference_generation/1(mag_ref)
  i_out_inverter_reference_pu/1 -> Manual Switch2/2
  u_out_inverter_pu/1 -> load_voltage_control/1(u_load)  "u_out_inverter_pu"
  u_out_inverter_reference_pu/1 -> load_voltage_control/2(u_load_reference)  "u_out_inverter_reference_pu"
  load_voltage_control/1(i_ref_internal) -> Manual Switch2/1

== system three_phase_dab/inverter_modA/single_phase_pll/double_integrator_observer ==
  theta : Inport
  Gain : Gain  Gain=Ldrso  Multiplication=Matrix(K*u)
  Gain1 : Gain  Gain=Adrso  Multiplication=Matrix(K*u)
  Gain2 : Gain  Gain=Crso  Multiplication=Matrix(K*u)
  Sum : Sum  Inputs=-+|
  Sum1 : Sum  Inputs=|++
  Unit Delay : UnitDelay  SampleTime=ts_inv  HasFrameUpgradeWarning=on
  Zero-Order Hold : ZeroOrderHold  SampleTime=ts_inv
  bounder1 : MATLAB Function  TreatAsAtomicUnit=on  SystemSampleTime=ts_inv
  bounder2 : MATLAB Function  TreatAsAtomicUnit=on  SystemSampleTime=ts_inv
  theta_hat : Outport
  wires:
  Gain/1 -> Sum1/1
  Gain2/1 -> bounder2/1(u)  "theta_hat"
  Gain1/1 -> Sum1/2
  Sum1/1 -> Unit Delay/1
  Sum/1 -> bounder1/1(u)  "e"
  Unit Delay/1 -> Gain1/1, Gain2/1
  theta/1 -> Zero-Order Hold/1  "theta"
  Zero-Order Hold/1 -> Sum/2  "theta_dsp"
  bounder1/1(y) -> Gain/1  "e_bounded"
  bounder2/1(y) -> theta_hat/1, Sum/1  "theta_hat_bounded"

== system three_phase_dab/inverter_modA/single_phase_pll/pi-ctrl ==
  x : Inport
  xref : Inport  Port=2
  1/Ti : Gain  Gain=kp  SaturateOnIntegerOverflow=on  OutDataTypeStr=Inherit: Same as input  ParamDataTypeStr=Inherit: Same as input
  Saturation : Saturate  UpperLimit=sat_pos  LowerLimit=sat_neg
  Sum1 : Sum  Inputs=+++  SaturateOnIntegerOverflow=on
  Sum2 : Sum  Inputs=-+  SaturateOnIntegerOverflow=on
  Sum3 : Sum  Inputs=-+  SaturateOnIntegerOverflow=on
  Unit Delay1 : UnitDelay  SampleTime=ts  HasFrameUpgradeWarning=on
  Unit Delay2 : UnitDelay  SampleTime=ts  HasFrameUpgradeWarning=on
  Unit Delay4 : UnitDelay  SampleTime=ts  HasFrameUpgradeWarning=on
  kp : Gain  Gain=ki*ts  SaturateOnIntegerOverflow=on  OutDataTypeStr=Inherit: Same as input  ParamDataTypeStr=Inherit: Same as input
  u : Outport
  wires:
  Saturation/1 -> Sum3/2, u/1
  Unit Delay4/1 -> Sum1/3
  Sum1/1 -> Saturation/1
  x/1 -> Unit Delay1/1
  Sum3/1 -> Unit Delay4/1
  1/Ti/1 -> Sum3/1, Sum1/1
  Sum2/1 -> 1/Ti/1, kp/1
  kp/1 -> Sum1/2
  xref/1 -> Unit Delay2/1
  Unit Delay1/1 -> Sum2/1
  Unit Delay2/1 -> Sum2/2

== system three_phase_dab/dab_modA/battery/battery_system/LithiumIonBattery ==
  Current Sensor : fl_lib/Electrical/Electrical Sensors/Current Sensor
  Electrical Reference1 : fl_lib/Electrical/Electrical Elements/Electrical Reference
  PS-Simulink Converter4 : nesl_utility/PS-Simulink Converter  PhysicalDomain=network_engine_domain  SubClassName=ps_output  LeftPortType=input  RightPortType=output  PseudoPeriodic=off  Frequencies=[]  VectorFormat=1-D array  Unit=1  AffineConversion=off
  PS-Simulink Converter5 : nesl_utility/PS-Simulink Converter  PhysicalDomain=network_engine_domain  SubClassName=ps_output  LeftPortType=input  RightPortType=output  PseudoPeriodic=off  Frequencies=[]  VectorFormat=1-D array  Unit=V  AffineConversion=on
  SOC_estimator : Subsystem  Commented=on
  To Workspace1 : ToWorkspace  VariableName=idc_battery_sim  SampleTime=tc
      settings: MaxDataPoints=Nc
  To Workspace2 : ToWorkspace  VariableName=udc_battery_sim  SampleTime=tc
      settings: MaxDataPoints=Nc
  Unit Delay5 : UnitDelay  SampleTime=ts_dab  HasFrameUpgradeWarning=on
  Voltage Sensor : fl_lib/Electrical/Electrical Sensors/Voltage Sensor
  ibat/vdc : Scope  NumInputPorts=2
      settings: SampleTime=tc  ActiveDisplayYMinimum=-1320.0904644876443  ActiveDisplayYMaximum=5476.2315205150016  DataLoggingVariableName=ScopeData6
  lithium ion cell analytical ocv : Subsystem
  Uout+ : PMIOPort  Side=Right
  Uout- : PMIOPort  Port=2  Side=Right
  wires:
  PS-Simulink Converter5/1 -> Unit Delay5/1
  PS-Simulink Converter4/1 -> To Workspace1/1, ibat/vdc/1  "i batt"
  Unit Delay5/1 -> To Workspace2/1, [vdc]
  [vdc] -> ibat/vdc/2  "vdc"
  connections:
  Current Sensor/RConn1 -- PS-Simulink Converter4/LConn1
  Uout+/RConn1 -- Current Sensor/RConn2 -- Voltage Sensor/LConn1
  Voltage Sensor/RConn1 -- PS-Simulink Converter5/LConn1
  Voltage Sensor/RConn2 -- Electrical Reference1/LConn1 -- lithium ion cell analytical ocv/RConn2 -- Uout-/RConn1
  lithium ion cell analytical ocv/RConn1 -- Current Sensor/LConn1

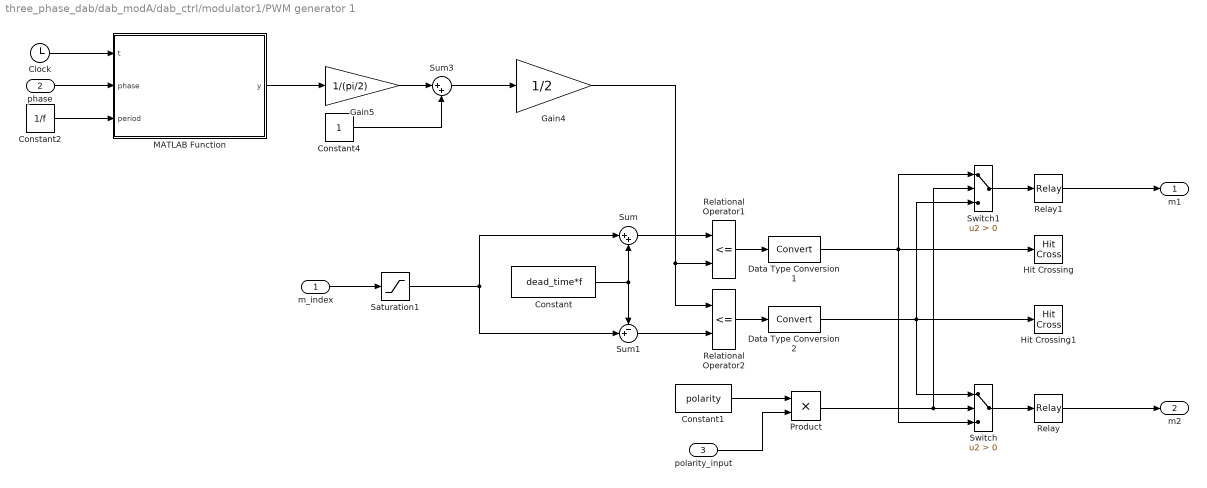
== system three_phase_dab/dab_modA/dab_ctrl/modulator1/PWM generator 1 ==
  m_index : Inport
  phase : Inport  Port=2
  polarity_input : Inport  Port=3
  Clock : Clock
  Constant : Constant  Value=dead_time*f
  Constant1 : Constant  Value=polarity
  Constant2 : Constant  Value=1/f
  Constant4 : Constant
  Data Type Conversion1 : DataTypeConversion
  Data Type Conversion2 : DataTypeConversion
  Gain4 : Gain  Gain=1/2
  Gain5 : Gain  Gain=1/(pi/2)
  Hit Crossing : HitCross  ShowOutputPort=off
  Hit Crossing1 : HitCross  ShowOutputPort=off
  MATLAB Function : MATLAB Function  TreatAsAtomicUnit=on
  Product : Product
  Relational Operator1 : RelationalOperator  Operator=<=  InputSameDT=off
  Relational Operator2 : RelationalOperator  Operator=<=  InputSameDT=off
  Relay : Relay  OnOutputValue=pos_cmd_gate  OffOutputValue=neg_cmd_gate
  Relay1 : Relay  OnOutputValue=pos_cmd_gate  OffOutputValue=neg_cmd_gate
  Saturation1 : Saturate  UpperLimit=m_up  LowerLimit=m_low
  Sum : Sum  Inputs=|++  SaturateOnIntegerOverflow=on
  Sum1 : Sum  Inputs=-+|  SaturateOnIntegerOverflow=on
  Sum3 : Sum  Inputs=|++
  Switch : Switch  Criteria=u2 > Threshold  SaturateOnIntegerOverflow=off  InputSameDT=off
  Switch1 : Switch  Criteria=u2 > Threshold  SaturateOnIntegerOverflow=off  InputSameDT=off
  m1 : Outport
  m2 : Outport  Port=2
  wires:
  Relational Operator1/1 -> Data Type Conversion1/1
  m_index/1 -> Saturation1/1
  Relational Operator2/1 -> Data Type Conversion2/1
  Data Type Conversion2/1 -> Switch/1, Switch1/3, Hit Crossing1/1
  Constant/1 -> Sum/2, Sum1/1
  Saturation1/1 -> Sum/1, Sum1/2
  Sum/1 -> Relational Operator1/1
  Sum1/1 -> Relational Operator2/2
  Gain4/1 -> Relational Operator2/1, Relational Operator1/2
  Data Type Conversion1/1 -> Hit Crossing/1, Switch/3, Switch1/1
  Switch/1 -> Relay/1
  Clock/1 -> MATLAB Function/1(t)
  Constant2/1 -> MATLAB Function/3(period)
  phase/1 -> MATLAB Function/2(phase)
  MATLAB Function/1(y) -> Gain5/1
  Gain5/1 -> Sum3/1
  Sum3/1 -> Gain4/1
  Constant4/1 -> Sum3/2
  Relay/1 -> m2/1
  Product/1 -> Switch1/2, Switch/2
  Switch1/1 -> Relay1/1
  Relay1/1 -> m1/1
  Constant1/1 -> Product/1
  polarity_input/1 -> Product/2

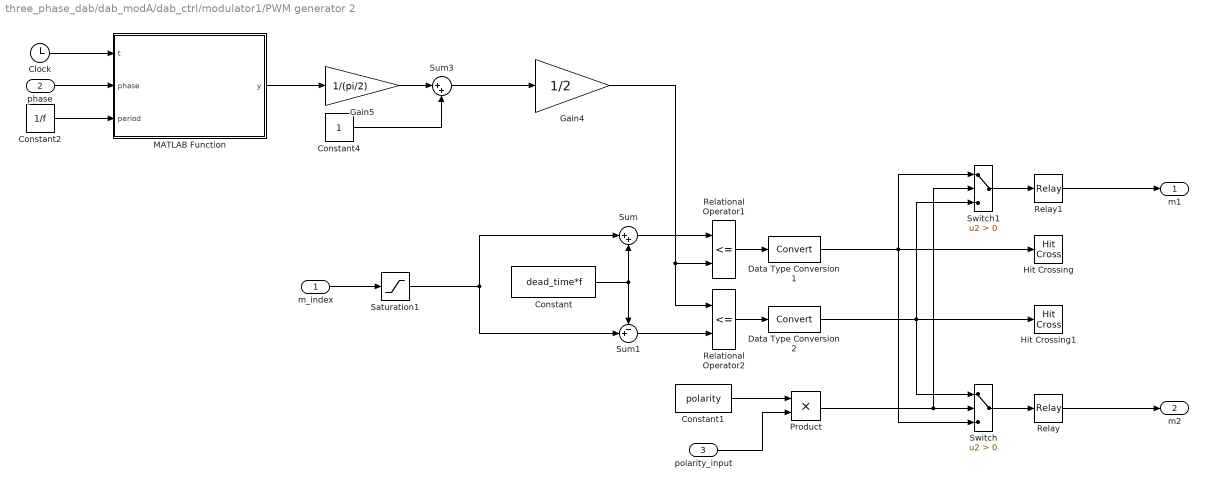
== system three_phase_dab/dab_modA/dab_ctrl/modulator1/PWM generator 2 ==
  m_index : Inport
  phase : Inport  Port=2
  polarity_input : Inport  Port=3
  Clock : Clock
  Constant : Constant  Value=dead_time*f
  Constant1 : Constant  Value=polarity
  Constant2 : Constant  Value=1/f
  Constant4 : Constant
  Data Type Conversion1 : DataTypeConversion
  Data Type Conversion2 : DataTypeConversion
  Gain4 : Gain  Gain=1/2
  Gain5 : Gain  Gain=1/(pi/2)
  Hit Crossing : HitCross  ShowOutputPort=off
  Hit Crossing1 : HitCross  ShowOutputPort=off
  MATLAB Function : MATLAB Function  TreatAsAtomicUnit=on
  Product : Product
  Relational Operator1 : RelationalOperator  Operator=<=  InputSameDT=off
  Relational Operator2 : RelationalOperator  Operator=<=  InputSameDT=off
  Relay : Relay  OnOutputValue=pos_cmd_gate  OffOutputValue=neg_cmd_gate
  Relay1 : Relay  OnOutputValue=pos_cmd_gate  OffOutputValue=neg_cmd_gate
  Saturation1 : Saturate  UpperLimit=m_up  LowerLimit=m_low
  Sum : Sum  Inputs=|++  SaturateOnIntegerOverflow=on
  Sum1 : Sum  Inputs=-+|  SaturateOnIntegerOverflow=on
  Sum3 : Sum  Inputs=|++
  Switch : Switch  Criteria=u2 > Threshold  SaturateOnIntegerOverflow=off  InputSameDT=off
  Switch1 : Switch  Criteria=u2 > Threshold  SaturateOnIntegerOverflow=off  InputSameDT=off
  m1 : Outport
  m2 : Outport  Port=2
  wires:
  polarity_input/1 -> Product/2
  Constant1/1 -> Product/1
  Relay1/1 -> m1/1
  Switch1/1 -> Relay1/1
  Product/1 -> Switch/2, Switch1/2
  Relay/1 -> m2/1
  Constant4/1 -> Sum3/2
  Sum3/1 -> Gain4/1
  Gain5/1 -> Sum3/1
  MATLAB Function/1(y) -> Gain5/1
  phase/1 -> MATLAB Function/2(phase)
  Constant2/1 -> MATLAB Function/3(period)
  Clock/1 -> MATLAB Function/1(t)
  Switch/1 -> Relay/1
  Data Type Conversion1/1 -> Switch1/1, Switch/3, Hit Crossing/1
  Gain4/1 -> Relational Operator1/2, Relational Operator2/1
  Sum1/1 -> Relational Operator2/2
  Sum/1 -> Relational Operator1/1
  Saturation1/1 -> Sum1/2, Sum/1
  Constant/1 -> Sum1/1, Sum/2
  Data Type Conversion2/1 -> Hit Crossing1/1, Switch1/3, Switch/1
  Relational Operator2/1 -> Data Type Conversion2/1
  m_index/1 -> Saturation1/1
  Relational Operator1/1 -> Data Type Conversion1/1

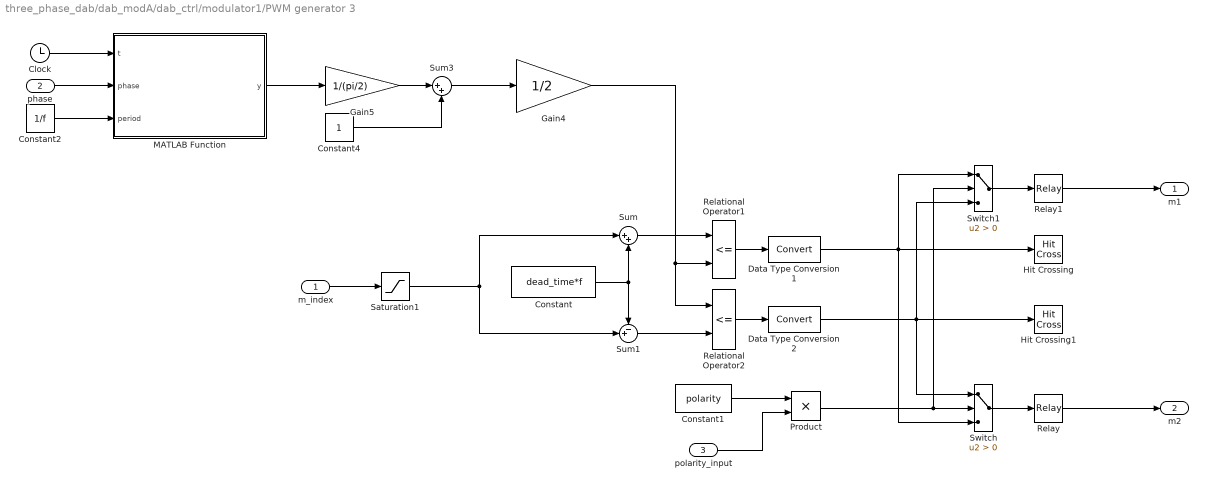
== system three_phase_dab/dab_modA/dab_ctrl/modulator1/PWM generator 3 ==
  m_index : Inport
  phase : Inport  Port=2
  polarity_input : Inport  Port=3
  Clock : Clock
  Constant : Constant  Value=dead_time*f
  Constant1 : Constant  Value=polarity
  Constant2 : Constant  Value=1/f
  Constant4 : Constant
  Data Type Conversion1 : DataTypeConversion
  Data Type Conversion2 : DataTypeConversion
  Gain4 : Gain  Gain=1/2
  Gain5 : Gain  Gain=1/(pi/2)
  Hit Crossing : HitCross  ShowOutputPort=off
  Hit Crossing1 : HitCross  ShowOutputPort=off
  MATLAB Function : MATLAB Function  TreatAsAtomicUnit=on
  Product : Product
  Relational Operator1 : RelationalOperator  Operator=<=  InputSameDT=off
  Relational Operator2 : RelationalOperator  Operator=<=  InputSameDT=off
  Relay : Relay  OnOutputValue=pos_cmd_gate  OffOutputValue=neg_cmd_gate
  Relay1 : Relay  OnOutputValue=pos_cmd_gate  OffOutputValue=neg_cmd_gate
  Saturation1 : Saturate  UpperLimit=m_up  LowerLimit=m_low
  Sum : Sum  Inputs=|++  SaturateOnIntegerOverflow=on
  Sum1 : Sum  Inputs=-+|  SaturateOnIntegerOverflow=on
  Sum3 : Sum  Inputs=|++
  Switch : Switch  Criteria=u2 > Threshold  SaturateOnIntegerOverflow=off  InputSameDT=off
  Switch1 : Switch  Criteria=u2 > Threshold  SaturateOnIntegerOverflow=off  InputSameDT=off
  m1 : Outport
  m2 : Outport  Port=2
  wires:
  polarity_input/1 -> Product/2
  Constant1/1 -> Product/1
  Relay1/1 -> m1/1
  Switch1/1 -> Relay1/1
  Product/1 -> Switch/2, Switch1/2
  Relay/1 -> m2/1
  Constant4/1 -> Sum3/2
  Sum3/1 -> Gain4/1
  Gain5/1 -> Sum3/1
  MATLAB Function/1(y) -> Gain5/1
  phase/1 -> MATLAB Function/2(phase)
  Constant2/1 -> MATLAB Function/3(period)
  Clock/1 -> MATLAB Function/1(t)
  Switch/1 -> Relay/1
  Data Type Conversion1/1 -> Switch1/1, Switch/3, Hit Crossing/1
  Gain4/1 -> Relational Operator1/2, Relational Operator2/1
  Sum1/1 -> Relational Operator2/2
  Sum/1 -> Relational Operator1/1
  Saturation1/1 -> Sum1/2, Sum/1
  Constant/1 -> Sum1/1, Sum/2
  Data Type Conversion2/1 -> Hit Crossing1/1, Switch1/3, Switch/1
  Relational Operator2/1 -> Data Type Conversion2/1
  m_index/1 -> Saturation1/1
  Relational Operator1/1 -> Data Type Conversion1/1

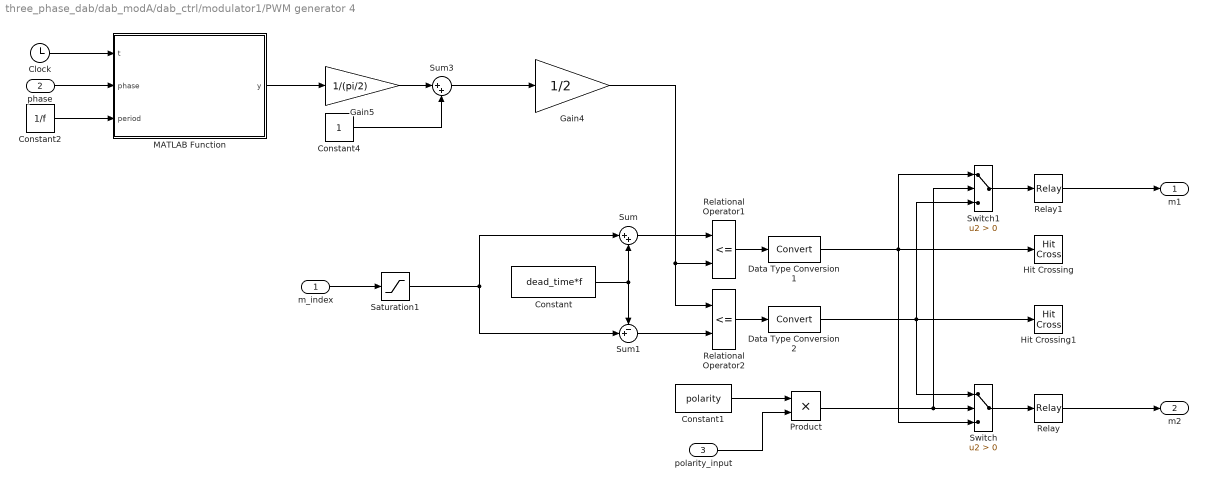
== system three_phase_dab/dab_modA/dab_ctrl/modulator1/PWM generator 4 ==
  m_index : Inport
  phase : Inport  Port=2
  polarity_input : Inport  Port=3
  Clock : Clock
  Constant : Constant  Value=dead_time*f
  Constant1 : Constant  Value=polarity
  Constant2 : Constant  Value=1/f
  Constant4 : Constant
  Data Type Conversion1 : DataTypeConversion
  Data Type Conversion2 : DataTypeConversion
  Gain4 : Gain  Gain=1/2
  Gain5 : Gain  Gain=1/(pi/2)
  Hit Crossing : HitCross  ShowOutputPort=off
  Hit Crossing1 : HitCross  ShowOutputPort=off
  MATLAB Function : MATLAB Function  TreatAsAtomicUnit=on
  Product : Product
  Relational Operator1 : RelationalOperator  Operator=<=  InputSameDT=off
  Relational Operator2 : RelationalOperator  Operator=<=  InputSameDT=off
  Relay : Relay  OnOutputValue=pos_cmd_gate  OffOutputValue=neg_cmd_gate
  Relay1 : Relay  OnOutputValue=pos_cmd_gate  OffOutputValue=neg_cmd_gate
  Saturation1 : Saturate  UpperLimit=m_up  LowerLimit=m_low
  Sum : Sum  Inputs=|++  SaturateOnIntegerOverflow=on
  Sum1 : Sum  Inputs=-+|  SaturateOnIntegerOverflow=on
  Sum3 : Sum  Inputs=|++
  Switch : Switch  Criteria=u2 > Threshold  SaturateOnIntegerOverflow=off  InputSameDT=off
  Switch1 : Switch  Criteria=u2 > Threshold  SaturateOnIntegerOverflow=off  InputSameDT=off
  m1 : Outport
  m2 : Outport  Port=2
  wires:
  Relational Operator1/1 -> Data Type Conversion1/1
  m_index/1 -> Saturation1/1
  Relational Operator2/1 -> Data Type Conversion2/1
  Data Type Conversion2/1 -> Switch/1, Switch1/3, Hit Crossing1/1
  Constant/1 -> Sum/2, Sum1/1
  Saturation1/1 -> Sum/1, Sum1/2
  Sum/1 -> Relational Operator1/1
  Sum1/1 -> Relational Operator2/2
  Gain4/1 -> Relational Operator2/1, Relational Operator1/2
  Data Type Conversion1/1 -> Hit Crossing/1, Switch/3, Switch1/1
  Switch/1 -> Relay/1
  Clock/1 -> MATLAB Function/1(t)
  Constant2/1 -> MATLAB Function/3(period)
  phase/1 -> MATLAB Function/2(phase)
  MATLAB Function/1(y) -> Gain5/1
  Gain5/1 -> Sum3/1
  Sum3/1 -> Gain4/1
  Constant4/1 -> Sum3/2
  Relay/1 -> m2/1
  Product/1 -> Switch1/2, Switch/2
  Switch1/1 -> Relay1/1
  Relay1/1 -> m1/1
  Constant1/1 -> Product/1
  polarity_input/1 -> Product/2

== system three_phase_dab/dab_modA/dab_ctrl/references/voltage_reference ==
  Constant1 : Constant  Value=Vout_dc_nom
  Rate Limiter : RateLimiter  RisingSlewLimit=Vout_dc_nom*10  FallingSlewLimit=-Vout_dc_nom*10  SampleTimeMode=inherited
  To Workspace2 : ToWorkspace  VariableName=vout_ref_modA_sim  SampleTime=ts_zvs
      settings: MaxDataPoints=Ns_zvs
  Vout_dc_nom : Step  Time=1e-3  After=Vout_dc_nom*1.15  SampleTime=0
  vout_ref : Outport
  wires:
  Vout_dc_nom/1 -> Rate Limiter/1
  Rate Limiter/1 -> To Workspace2/1, vout_ref/1

== system three_phase_dab/dab_modA/dab_ctrl/vi ctrl/Iout Ctrl ==
  iout_ref : Inport
  iout : Inport  Port=2
  Product : Product
  Rate Limiter : RateLimiter  FallingSlewLimit=0  SampleTimeMode=inherited
  Saturation1 : Saturate  UpperLimit=1  LowerLimit=0  OutDataTypeStr=double
  Step : Step  Time=0.1  SampleTime=0
  Sum2 : Sum  Inputs=+-  OutDataTypeStr=double  AccumDataTypeStr=double  SaturateOnIntegerOverflow=on
  To Workspace2 : ToWorkspace  VariableName=iout_ref_dsp_modA_sim  SampleTime=ts_zvs
      settings: MaxDataPoints=Ns_zvs
  To Workspace9 : ToWorkspace  VariableName=iout_dsp_modA_sim  SampleTime=ts_zvs
      settings: MaxDataPoints=Ns_zvs
  iout_ctrl : Subsystem
  ctrli_out : Outport
  wires:
  iout_ctrl/1(ctrli_out) -> ctrli_out/1
  iout/1 -> To Workspace9/1, Sum2/2
  iout_ref/1 -> Sum2/1, To Workspace2/1
  Rate Limiter/1 -> Saturation1/1
  Saturation1/1 -> Product/1
  Step/1 -> Rate Limiter/1
  Sum2/1 -> Product/2
  Product/1 -> iout_ctrl/1(i_tilde)

== system three_phase_dab/dab_modA/dab_ctrl/vi ctrl/Vout Ctrl ==
  vout_ref : Inport
  vout : Inport  Port=2
  Product : Product
  Rate Limiter : RateLimiter  FallingSlewLimit=0  SampleTimeMode=inherited
  Saturation1 : Saturate  UpperLimit=1  LowerLimit=0  OutDataTypeStr=double
  Step : Step  Time=0.1  SampleTime=0
  Sum2 : Sum  Inputs=+-  OutDataTypeStr=double  AccumDataTypeStr=double  SaturateOnIntegerOverflow=on
  To Workspace2 : ToWorkspace  VariableName=vout_ref_dsp_modA_sim  SampleTime=ts_zvs
      settings: MaxDataPoints=Ns_zvs
  To Workspace9 : ToWorkspace  VariableName=vout_dsp_modA_sim  SampleTime=ts_zvs
      settings: MaxDataPoints=Ns_zvs
  vout_ctrl : Subsystem
  ctrlv_out : Outport
  wires:
  vout_ref/1 -> To Workspace2/1, Sum2/1
  vout/1 -> To Workspace9/1, Sum2/2
  vout_ctrl/1(ctrlv_out) -> ctrlv_out/1
  Sum2/1 -> Product/2
  Product/1 -> vout_ctrl/1(ixi_tilde)
  Step/1 -> Rate Limiter/1
  Rate Limiter/1 -> Saturation1/1
  Saturation1/1 -> Product/1
